simulink model "sampleModel60"  (R2021b)
settings: Solver=VariableStepAuto  StartTime=0.0  StopTime=10.0  RelTol=1e-3
undefined symbols (not defined in the file or in its folder): DiscIntNeverNeededParam
libraries: simulink x12, slpidlib x2
settings Model: Creator=user  LastModifiedBy=user

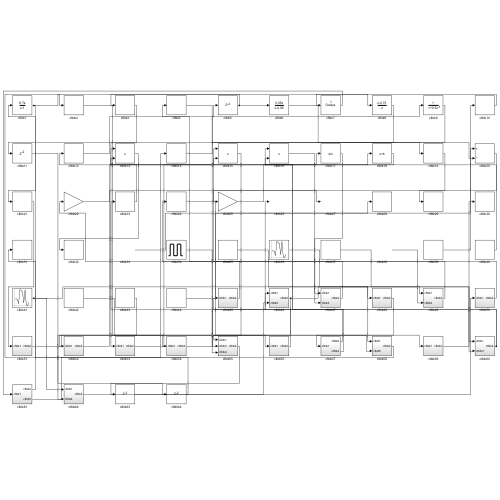
[thumbnail: Simulink's stored preview of the top-level diagram]
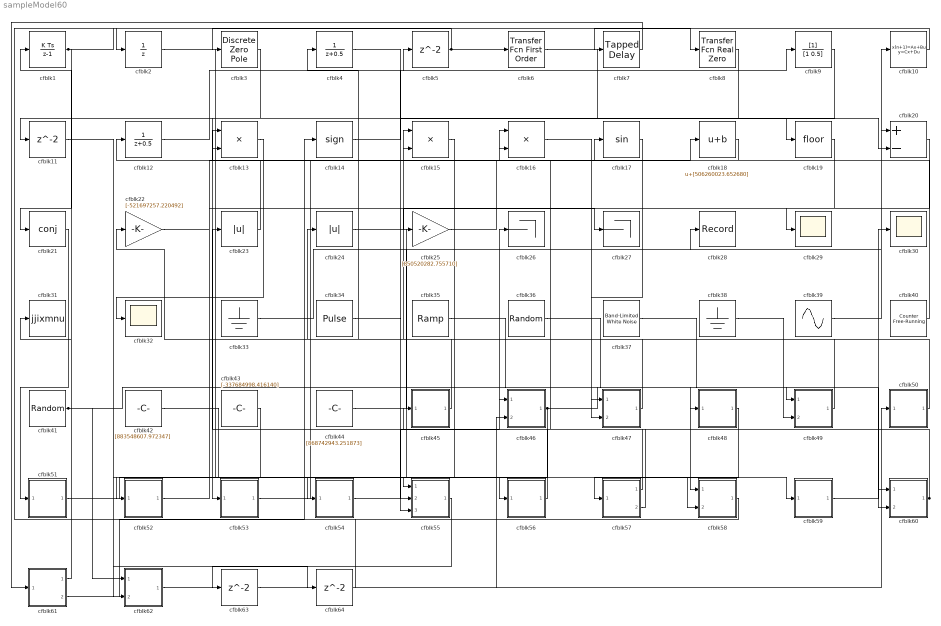
== system sampleModel60 ==
  cfblk1 : DiscreteIntegrator  ICPrevOutput=DiscIntNeverNeededParam  ICPrevScaledInput=DiscIntNeverNeededParam
  cfblk10 : DiscreteStateSpace
  cfblk{5,11,63..64} (4 alike) : Delay  SampleTime=1
  cfblk12 : DiscreteTransferFcn  SampleTime=1
  cfblk13 : Product  Inputs=**
  cfblk14 : Signum
  cfblk15 : Product
  cfblk16 : Product
  cfblk17 : Trigonometry
  cfblk18 : Bias  Bias=[506260023.652680]
  cfblk19 : Rounding
  cfblk2 : UnitDelay  HasFrameUpgradeWarning=on
  cfblk20 : Sum  Inputs=+-
  cfblk21 : Math  Operator=conj  SaturateOnIntegerOverflow=on
  cfblk22 : Gain  Gain=[-521697257.220492]
  cfblk23 : Abs
  cfblk24 : Abs
  cfblk25 : Gain  Gain=[850520282.755710]
  cfblk26 : Terminator
  cfblk27 : Terminator
  cfblk28 : Record  FileSettingsInternal="{\"entries\":[{\"content\":{\"excelSettings\":{\"content\":{},\"type\":\"Streamout.ExcelSettings\"}},\"type\":\"Streamout.FileSettingStorage\",\"uuid\":\"4c679408-955d-4ff0-bf7e-06dd5c5409d8\"}],\"packageUris\":[\"http://schema.mathworks.com/mf0/streamout_blocks/R2020a\"],\"version\":\"1.0\"}"  SignalsInternal="{\"entries\":[{\"content\":{\"signals\":[{\"content\":{\"blockPath\":[\"sampleModel60/cfblk28\"],\"channel\":[],\"dimensions\":[1],\"domain\":\"sampleModel60/cfblk28\",\"lineColor\":\"#4dbeee\",\"plots\":[1],\"port\":1,\"sid\":[\"\"],\"signalID\":2207,\"signalName\":\"cfblk44\"},\"type\":\"RecordBlkView.Signal\",\"uuid\":\"6fc09847-7afc-4846-a01f-61bfadea7150\"}]},\"type\":\"RecordBlkView.InputSignals\",\"uuid\":\"2313032d-359a-41a9-a05e-b1a7dad40221\"}],\"packageUris\":[\"http://schema.mathworks.com/mf0/streamout_blocks/R2020a\"],\"version\":\"1.0\"}"  VisualizationBindings="{\"sparklinesplugin\":{\"info\":[{\"bindingParametersList\":[],\"subplotID\":1}]}}"
  cfblk29 : Scope
  cfblk3 : DiscreteZeroPole  Poles=[0 0.5]  Gain=1
  cfblk30 : Scope
  cfblk31 : ToWorkspace  VariableName=jjixmnu  SaveFormat=Timeseries  SampleTime=-1
  cfblk32 : Scope
  cfblk33 : Ground
  cfblk34 : DiscretePulseGenerator  PulseType=Time based  Amplitude=[-729799359.660639]  Period=[20499576.336896]  PulseWidth=5  PhaseDelay=[2.000000]
  cfblk35 : simulink/Sources/Ramp  slope=[-9962.177894]  start=[43.030977]  InitialOutput=[-979981.461809]
  cfblk36 : RandomNumber  Mean=[-98263.089935]  Variance=[84048.525464]  Seed=[770043193.000000]  SampleTime=0.1
  cfblk37 : simulink/Sources/Band-Limited White Noise  Cov=[8571597638.096084]  Ts=0.1  seed=[9334520980.000000]
  cfblk38 : Ground
  cfblk39 : Sin  Amplitude=[-969853810.219643]  Bias=[-620311576.085574]  SampleTime=0
  cfblk4 : DiscreteTransferFcn  SampleTime=1
  cfblk40 : simulink/Sources/Counter Free-Running  NumBits=[41.000000]  tsamp=-1
  cfblk41 : RandomNumber  Mean=[95459.502564]  Variance=[57526.067039]  Seed=[562370184.000000]  SampleTime=0.1
  cfblk42 : Constant  Value=[883548607.972347]  SampleTime=1
  cfblk43 : Constant  Value=[-337684998.416140]  SampleTime=1
  cfblk44 : Constant  Value=[868742943.251873]  SampleTime=1
  cfblk45 : Subsystem
  cfblk46 : Subsystem
  cfblk47 : Subsystem
  cfblk48 : Subsystem
  cfblk49 : Subsystem
  cfblk50 : Subsystem
  cfblk51 : Subsystem
  cfblk52 : Subsystem
  cfblk53 : Subsystem
  cfblk54 : Subsystem
  cfblk55 : Subsystem
  cfblk56 : Subsystem
  cfblk57 : Subsystem
  cfblk58 : Subsystem
  cfblk59 : Subsystem
  cfblk6 : simulink/Discrete/Transfer Fcn First Order  PoleZ=0.95  ICPrevOutput=0.0  DoSatur=off
  cfblk60 : Subsystem
  cfblk61 : Subsystem
  cfblk62 : Subsystem
  cfblk7 : simulink/Discrete/Tapped Delay  vinit=0.0  samptime=-1  NumDelays=1  DelayOrder=Oldest  includeCurrent=off
  cfblk8 : simulink/Discrete/Transfer Fcn Real Zero  ZeroZ=0.75  ICPrevInput=0.0  DoSatur=off
      settings: SourceProductBaseCode=SL
  cfblk9 : DiscreteFilter  SampleTime=1
  wires:
  cfblk21/1 -> cfblk51/1(cfblk1)
  cfblk23/1 -> cfblk12/1
  cfblk33/1 -> cfblk10/1
  cfblk13/1 -> cfblk32/1
  cfblk48/1(cfblk2) -> cfblk57/1(cfblk1)
  cfblk53/1(cfblk2) -> cfblk17/1
  cfblk45/1(cfblk2) -> cfblk24/1
  cfblk49/1(cfblk2) -> cfblk15/1
  cfblk46/1(cfblk2) -> cfblk49/1(cfblk1), cfblk62/2(cfblk4)
  cfblk8/1 -> cfblk11/1
  cfblk44/1 -> cfblk28/1
  cfblk62/1(cfblk2) -> cfblk50/1(cfblk1)
  cfblk14/1 -> cfblk9/1
  cfblk6/1 -> cfblk19/1
  cfblk39/1 -> cfblk20/1
  cfblk57/1(cfblk2) -> cfblk26/1
  cfblk5/1 -> cfblk6/1, cfblk3/1
  cfblk47/1(cfblk2) -> cfblk22/1
  cfblk2/1 -> cfblk59/1(cfblk1)
  cfblk60/1(cfblk2) -> cfblk16/1, cfblk16/2
  cfblk3/1 -> cfblk53/1(cfblk1)
  cfblk58/1(cfblk2) -> cfblk2/1
  cfblk1/1 -> cfblk21/1, cfblk8/1
  cfblk59/1(cfblk2) -> cfblk30/1
  cfblk7/1 -> cfblk61/1(cfblk1)
  cfblk36/1 -> cfblk58/1(cfblk1)
  cfblk40/1 -> cfblk13/1
  cfblk24/1 -> cfblk56/1(cfblk1)
  cfblk37/1 -> cfblk60/1(cfblk1)
  cfblk51/1(cfblk2) -> cfblk54/1(cfblk1)
  cfblk57/2(cfblk4) -> cfblk45/1(cfblk1)
  cfblk16/1 -> cfblk47/1(cfblk1)
  cfblk17/1 -> cfblk47/2(cfblk3)
  cfblk20/1 -> cfblk25/1
  cfblk61/1(cfblk2) -> cfblk31/1
  cfblk43/1 -> cfblk52/1(cfblk1)
  cfblk15/1 -> cfblk55/1(cfblk1)
  cfblk25/1 -> cfblk18/1
  cfblk19/1 -> cfblk29/1
  cfblk54/1(cfblk2) -> cfblk46/1(cfblk1)
  cfblk42/1 -> cfblk58/2(cfblk5)
  cfblk10/1 -> cfblk7/1
  cfblk52/1(cfblk2) -> cfblk15/2
  cfblk38/1 -> cfblk49/2(cfblk4)
  cfblk12/1 -> cfblk5/1
  cfblk35/1 -> cfblk60/2(cfblk3)
  cfblk4/1 -> cfblk20/2
  cfblk41/1 -> cfblk48/1(cfblk1), cfblk62/1(cfblk1)
  cfblk61/2(cfblk5) -> cfblk14/1
  cfblk18/1 -> cfblk13/2
  cfblk56/1(cfblk2) -> cfblk23/1
  cfblk22/1 -> cfblk27/1
  cfblk50/1(cfblk2) -> cfblk4/1
  cfblk9/1 -> cfblk55/2(cfblk3)
  cfblk34/1 -> cfblk55/3(cfblk4)
  cfblk55/1(cfblk2) -> cfblk63/1
  cfblk63/1 -> cfblk46/2(cfblk3)
  cfblk11/1 -> cfblk64/1
  cfblk64/1 -> cfblk1/1

== system sampleModel60/cfblk45 ==
  cfblk1 : Inport
  cfblk3 : Rounding
  cfblk2 : Outport
  wires:
  cfblk1/1 -> cfblk3/1
  cfblk3/1 -> cfblk2/1

== system sampleModel60/cfblk46 ==
  cfblk1 : Inport
  cfblk3 : Inport  Port=2
  cfblk2 : Outport
  wires:
  cfblk1/1 -> cfblk2/1

== system sampleModel60/cfblk47 ==
  cfblk1 : Inport
  cfblk3 : Inport  Port=2
  cfblk2 : Outport
  wires:
  cfblk1/1 -> cfblk2/1

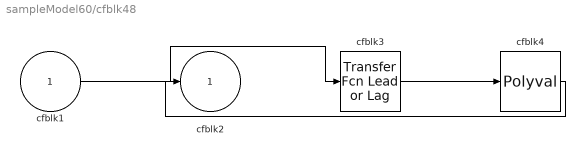
== system sampleModel60/cfblk48 ==
  cfblk1 : Inport
  cfblk3 : simulink/Discrete/Transfer Fcn Lead or Lag  PoleZ=0.95  ZeroZ=0.75  ICPrevOutput=0.0  ICPrevInput=0.0  DoSatur=off
      settings: SourceProductBaseCode=SL
  cfblk4 : Polyval  Coefs=[ +2.081618890e-019, -1.441693666e-014, +4.719686976e-010, -8.536869453e-006, +1.621573104e-001, -8.087801117e+001 ]
  cfblk2 : Outport
  wires:
  cfblk1/1 -> cfblk3/1
  cfblk3/1 -> cfblk4/1
  cfblk4/1 -> cfblk2/1

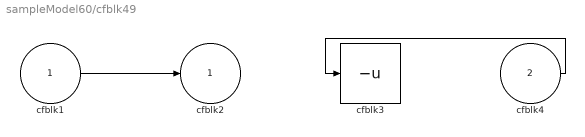
== system sampleModel60/cfblk49 ==
  cfblk1 : Inport
  cfblk4 : Inport  Port=2
  cfblk3 : UnaryMinus
  cfblk2 : Outport
  wires:
  cfblk4/1 -> cfblk3/1
  cfblk1/1 -> cfblk2/1

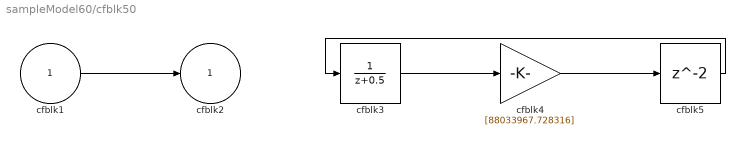
== system sampleModel60/cfblk50 ==
  cfblk1 : Inport
  cfblk3 : DiscreteTransferFcn  SampleTime=1
  cfblk4 : Gain  Gain=[88033967.728316]
  cfblk5 : Delay  SampleTime=1
  cfblk2 : Outport
  wires:
  cfblk1/1 -> cfblk2/1
  cfblk3/1 -> cfblk4/1
  cfblk4/1 -> cfblk5/1
  cfblk5/1 -> cfblk3/1

== system sampleModel60/cfblk51 ==
  cfblk1 : Inport
  cfblk3 : DiscreteStateSpace
  cfblk2 : Outport
  wires:
  cfblk1/1 -> cfblk2/1, cfblk3/1

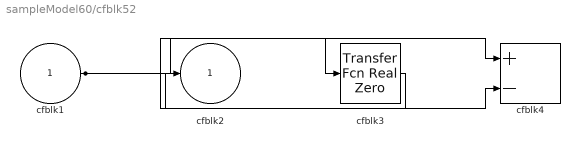
== system sampleModel60/cfblk52 ==
  cfblk1 : Inport
  cfblk3 : simulink/Discrete/Transfer Fcn Real Zero  ZeroZ=0.75  ICPrevInput=0.0  DoSatur=off
      settings: SourceProductBaseCode=SL
  cfblk4 : Sum  Inputs=+-
  cfblk2 : Outport
  wires:
  cfblk1/1 -> cfblk3/1, cfblk4/1, cfblk4/2
  cfblk3/1 -> cfblk2/1

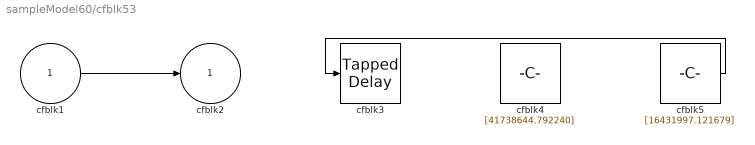
== system sampleModel60/cfblk53 ==
  cfblk1 : Inport
  cfblk3 : simulink/Discrete/Tapped Delay  vinit=0.0  samptime=-1  NumDelays=1  DelayOrder=Oldest  includeCurrent=off
  cfblk4 : Constant  Value=[41738644.792240]  SampleTime=1
  cfblk5 : Constant  Value=[16431997.121679]  SampleTime=1
  cfblk2 : Outport
  wires:
  cfblk5/1 -> cfblk3/1
  cfblk1/1 -> cfblk2/1

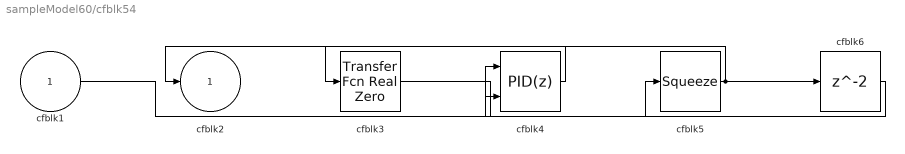
== system sampleModel60/cfblk54 ==
  cfblk1 : Inport
  cfblk3 : simulink/Discrete/Transfer Fcn Real Zero  ZeroZ=0.75  ICPrevInput=0.0  DoSatur=off
      settings: SourceProductBaseCode=SL
  cfblk4 : slpidlib/PID Controller (2DOF)  Controller=PID  Form=Parallel  TimeDomain=Discrete-time  UseExternalTs=off  SampleTime=1  IntegratorMethod=Forward Euler  FilterMethod=Forward Euler  ControllerParametersSource=internal  P=1  I=1  D=0  UseFilter=on  N=100  b=1  c=1  TunerSelectOption=Transfer Function Based (PID Tuner App)  InitialConditionSource=internal  InitialConditionForIntegrator=0  InitialConditionForFilter=0  DifferentiatorICPrevScaledInput=0  ExternalReset=none  TrackingMode=off  Kt=1  LimitOutput=off  SatLimitsSource=internal  UpperSaturationLimit=inf  LowerSaturationLimit=-inf  LinearizeAsGain=off  AntiWindupMode=none  Kb=1  POutMin=[]  POutMax=[]  IOutMin=[]  IOutMax=[]  DOutMin=[]  DOutMax=[]  NOutMin=[]  NOutMax=[]  bOutMin=[]  bOutMax=[]  cOutMin=[]  cOutMax=[]  SumOutMin=[]  SumOutMax=[]  SaturationOutMin=[]  SaturationOutMax=[]  PParamMin=[]  PParamMax=[]  IParamMin=[]  IParamMax=[]  DParamMin=[]  DParamMax=[]  NParamMin=[]  NParamMax=[]  bParamMin=[]  bParamMax=[]  cParamMin=[]  cParamMax=[]  KbParamMin=[]  KbParamMax=[]  KtParamMin=[]  KtParamMax=[]  KbOutMin=[]  KbOutMax=[]  KtOutMin=[]  KtOutMax=[]  IntegratorOutMin=[]  IntegratorOutMax=[]  FilterOutMin=[]  FilterOutMax=[]  SumI1OutMin=[]  SumI1OutMax=[]  SumI2OutMin=[]  SumI2OutMax=[]  SumI3OutMin=[]  SumI3OutMax=[]  SumI4OutMin=[]  SumI4OutMax=[]  SumDOutMin=[]  SumDOutMax=[]  Sum1OutMin=[]  Sum1OutMax=[]  Sum2OutMin=[]  Sum2OutMax=[]  Sum3OutMin=[]  Sum3OutMax=[]  DifferentiatorOutMin=[]  DifferentiatorOutMax=[]  FilterDiffOutCoefMin=[]  FilterDiffOutCoefMax=[]  ReciprocalOutMin=[]  ReciprocalOutMax=[]  SumDenOutMin=[]  SumDenOutMax=[]  SumNumOutMin=[]  SumNumOutMax=[]  DivideOutMin=[]  DivideOutMax=[]  UdiffTsProdOutMin=[]  UdiffTsProdOutMax=[]  NTsProdOutMin=[]  NTsProdOutMax=[]  UintegralTsProdOutMin=[]  UintegralTsProdOutMax=[]  UngainTsProdOutMin=[]  UngainTsProdOutMax=[]  IntegratorContinuousStateAttributes=''  IntegratorStateMustResolveToSignalObject=off  IntegratorRTWStateStorageClass=Auto  FilterContinuousStateAttributes=''  FilterStateMustResolveToSignalObject=off  FilterRTWStateStorageClass=Auto  ParallelPVariant=InternalParameters  IdealPVariant=Disabled  IVariant=InternalParameters  DVariant=InternalParameters  bVariant=InternalParameters  cVariant=InternalParameters  IntegratorVariant=Discrete  SatVariant=Disabled  AWVariant=Passthrough  PCopyVariant=Disabled  TRVariant=Disabled  FdbkBlocksVariant=Forward  IdealPFdbkVariant=Disabled  SatFdbkVariant=Disabled  DerivativeFilterVariant=ForwardEulerFilter  NVariant=InternalParameters  NCopyVariant=Disabled  FilterICVariant=InternalICsFilter  IntegratorICVariant=InternalICs  ExternalResetVariant=Disabled  TRSumVariant=Passthrough  SumFdbkVariant=Disabled  SumVariant=Sum_PID  TsampFilterVariant=InternalTs  TsampNgainVariant=Passthrough  TsampIntegralVariant=Passthrough  ExternalSaturationOutDataTypeStr=Inherit: Same as second input
      settings: SourceProductBaseCode=SL
  cfblk5 : Squeeze
  cfblk6 : Delay  SampleTime=1
  cfblk2 : Outport
  wires:
  cfblk5/1 -> cfblk2/1, cfblk6/1
  cfblk1/1 -> cfblk4/1
  cfblk4/1 -> cfblk3/1
  cfblk3/1 -> cfblk5/1
  cfblk6/1 -> cfblk4/2

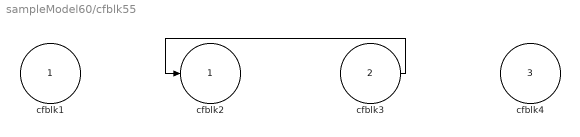
== system sampleModel60/cfblk55 ==
  cfblk1 : Inport
  cfblk3 : Inport  Port=2
  cfblk4 : Inport  Port=3
  cfblk2 : Outport
  wires:
  cfblk3/1 -> cfblk2/1

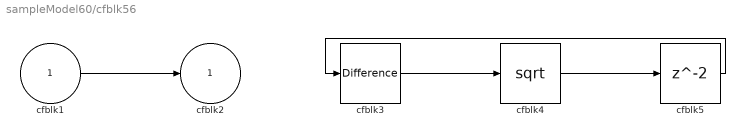
== system sampleModel60/cfblk56 ==
  cfblk1 : Inport
  cfblk3 : simulink/Discrete/Difference  ICPrevInput=0.0  OutMin=[]  OutMax=[]  OutDataTypeStr=Inherit: Inherit via back propagation  OutDataType=fixdt(1, 16)  OutScaling=2^-10  DoSatur=off
  cfblk4 : Sqrt  SaturateOnIntegerOverflow=on
  cfblk5 : Delay  SampleTime=1
  cfblk2 : Outport
  wires:
  cfblk1/1 -> cfblk2/1
  cfblk3/1 -> cfblk4/1
  cfblk4/1 -> cfblk5/1
  cfblk5/1 -> cfblk3/1

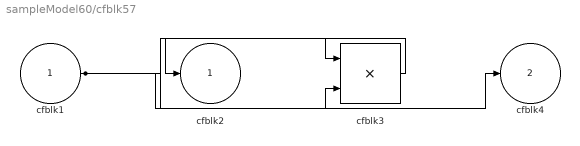
== system sampleModel60/cfblk57 ==
  cfblk1 : Inport
  cfblk3 : Product
  cfblk2 : Outport
  cfblk4 : Outport  Port=2
  wires:
  cfblk3/1 -> cfblk2/1
  cfblk1/1 -> cfblk4/1, cfblk3/1, cfblk3/2

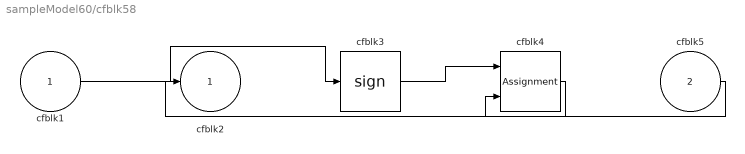
== system sampleModel60/cfblk58 ==
  cfblk1 : Inport
  cfblk5 : Inport  Port=2
  cfblk3 : Signum
  cfblk4 : Assignment  DiagnosticForDimensions=Warning  IndexOptions=Index vector (dialog)  Indices=1  OutputSizes=1
  cfblk2 : Outport
  wires:
  cfblk1/1 -> cfblk3/1
  cfblk4/1 -> cfblk2/1
  cfblk3/1 -> cfblk4/1
  cfblk5/1 -> cfblk4/2

== system sampleModel60/cfblk59 ==
  cfblk1 : Inport
  cfblk3 : Constant  Value=[-340004320.637826]  SampleTime=1
  cfblk2 : Outport
  wires:
  cfblk1/1 -> cfblk2/1

== system sampleModel60/cfblk60 ==
  cfblk1 : Inport
  cfblk3 : Inport  Port=2
  cfblk2 : Outport
  wires:
  cfblk3/1 -> cfblk2/1

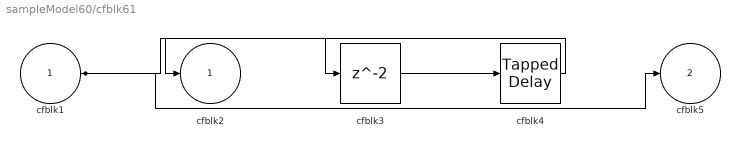
== system sampleModel60/cfblk61 ==
  cfblk1 : Inport
  cfblk3 : Delay  SampleTime=1
  cfblk4 : simulink/Discrete/Tapped Delay  vinit=0.0  samptime=-1  NumDelays=1  DelayOrder=Oldest  includeCurrent=off
  cfblk2 : Outport
  cfblk5 : Outport  Port=2
  wires:
  cfblk3/1 -> cfblk4/1
  cfblk4/1 -> cfblk2/1
  cfblk1/1 -> cfblk5/1, cfblk3/1

== system sampleModel60/cfblk62 ==
  cfblk1 : Inport
  cfblk4 : Inport  Port=2
  cfblk3 : slpidlib/PID Controller (2DOF)  Controller=PID  Form=Parallel  TimeDomain=Discrete-time  UseExternalTs=off  SampleTime=1  IntegratorMethod=Forward Euler  FilterMethod=Forward Euler  ControllerParametersSource=internal  P=1  I=1  D=0  UseFilter=on  N=100  b=1  c=1  TunerSelectOption=Transfer Function Based (PID Tuner App)  InitialConditionSource=internal  InitialConditionForIntegrator=0  InitialConditionForFilter=0  DifferentiatorICPrevScaledInput=0  ExternalReset=none  TrackingMode=off  Kt=1  LimitOutput=off  SatLimitsSource=internal  UpperSaturationLimit=inf  LowerSaturationLimit=-inf  LinearizeAsGain=off  AntiWindupMode=none  Kb=1  POutMin=[]  POutMax=[]  IOutMin=[]  IOutMax=[]  DOutMin=[]  DOutMax=[]  NOutMin=[]  NOutMax=[]  bOutMin=[]  bOutMax=[]  cOutMin=[]  cOutMax=[]  SumOutMin=[]  SumOutMax=[]  SaturationOutMin=[]  SaturationOutMax=[]  PParamMin=[]  PParamMax=[]  IParamMin=[]  IParamMax=[]  DParamMin=[]  DParamMax=[]  NParamMin=[]  NParamMax=[]  bParamMin=[]  bParamMax=[]  cParamMin=[]  cParamMax=[]  KbParamMin=[]  KbParamMax=[]  KtParamMin=[]  KtParamMax=[]  KbOutMin=[]  KbOutMax=[]  KtOutMin=[]  KtOutMax=[]  IntegratorOutMin=[]  IntegratorOutMax=[]  FilterOutMin=[]  FilterOutMax=[]  SumI1OutMin=[]  SumI1OutMax=[]  SumI2OutMin=[]  SumI2OutMax=[]  SumI3OutMin=[]  SumI3OutMax=[]  SumI4OutMin=[]  SumI4OutMax=[]  SumDOutMin=[]  SumDOutMax=[]  Sum1OutMin=[]  Sum1OutMax=[]  Sum2OutMin=[]  Sum2OutMax=[]  Sum3OutMin=[]  Sum3OutMax=[]  DifferentiatorOutMin=[]  DifferentiatorOutMax=[]  FilterDiffOutCoefMin=[]  FilterDiffOutCoefMax=[]  ReciprocalOutMin=[]  ReciprocalOutMax=[]  SumDenOutMin=[]  SumDenOutMax=[]  SumNumOutMin=[]  SumNumOutMax=[]  DivideOutMin=[]  DivideOutMax=[]  UdiffTsProdOutMin=[]  UdiffTsProdOutMax=[]  NTsProdOutMin=[]  NTsProdOutMax=[]  UintegralTsProdOutMin=[]  UintegralTsProdOutMax=[]  UngainTsProdOutMin=[]  UngainTsProdOutMax=[]  IntegratorContinuousStateAttributes=''  IntegratorStateMustResolveToSignalObject=off  IntegratorRTWStateStorageClass=Auto  FilterContinuousStateAttributes=''  FilterStateMustResolveToSignalObject=off  FilterRTWStateStorageClass=Auto  ParallelPVariant=InternalParameters  IdealPVariant=Disabled  IVariant=InternalParameters  DVariant=InternalParameters  bVariant=InternalParameters  cVariant=InternalParameters  IntegratorVariant=Discrete  SatVariant=Disabled  AWVariant=Passthrough  PCopyVariant=Disabled  TRVariant=Disabled  FdbkBlocksVariant=Forward  IdealPFdbkVariant=Disabled  SatFdbkVariant=Disabled  DerivativeFilterVariant=ForwardEulerFilter  NVariant=InternalParameters  NCopyVariant=Disabled  FilterICVariant=InternalICsFilter  IntegratorICVariant=InternalICs  ExternalResetVariant=Disabled  TRSumVariant=Passthrough  SumFdbkVariant=Disabled  SumVariant=Sum_PID  TsampFilterVariant=InternalTs  TsampNgainVariant=Passthrough  TsampIntegralVariant=Passthrough  ExternalSaturationOutDataTypeStr=Inherit: Same as second input
      settings: SourceProductBaseCode=SL
  cfblk2 : Outport
  wires:
  cfblk3/1 -> cfblk2/1
  cfblk4/1 -> cfblk3/1
  cfblk1/1 -> cfblk3/2
